simulink model "r22_05"  (Simulink 8.6)
settings: Solver=FixedStepDiscrete  StartTime=0.0  StopTime=500  FixedStep=0.1  RelTol=1e-3
undefined symbols (not defined in the file or in its folder): sldvsubsys
libraries: simulink x13, sldvlib x2
settings Model: Creator=Kerianne  LastModifiedBy=mike
settings DataIOCC: SignalLogging=off
settings OptimizationCC: DefaultParameterBehavior=Inlined
settings DebuggingCC: MultiTaskDSMMsg=warning  MultiTaskCondExecSysMsg=none  FcnCallInpInsideContextMsg=EnableAllAsError
settings GRTTargetCC: CombineOutputUpdateFcns=on  GRTInterface=off
settings ConfigComp: DVTestSuiteOptimization=CombinedObjectives (Nonlinear Extended)

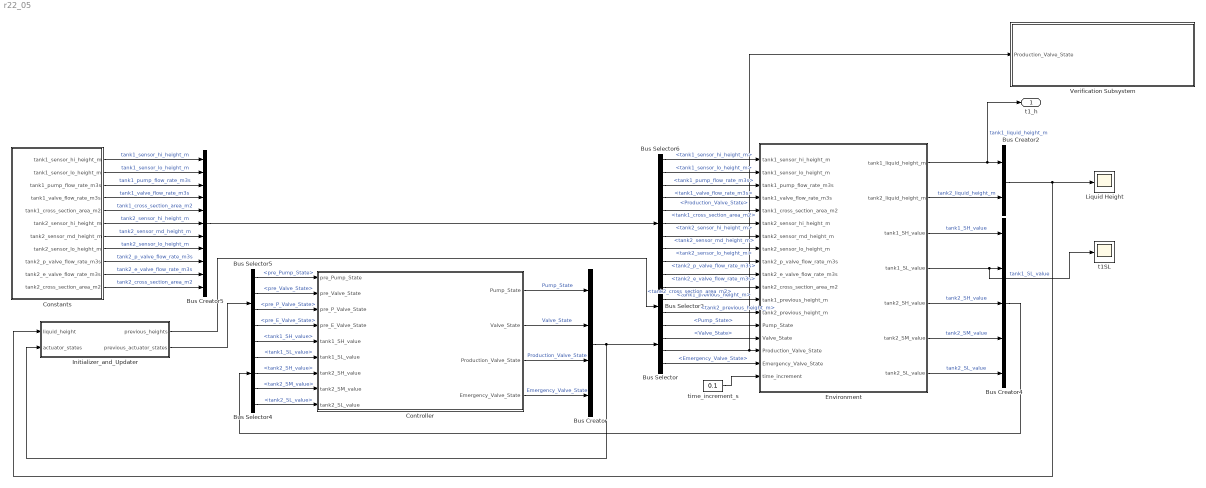
== system r22_05 ==
  Bus Creator : BusCreator  Inputs=4
  Bus Creator2 : BusCreator  Inputs='tank1_liquid_height_m','tank2_liquid_height_m'
  Bus Creator4 : BusCreator  Inputs='tank1_SH_value','tank1_SL_value','tank2_SH_value','tank2_SM_value','tank2_SL_value'
  Bus Creator5 : BusCreator  Inputs='tank1_sensor_hi_height_m','tank1_sensor_lo_height_m','tank1_pump_flow_rate_m3s','tank1_valve_flow_rate_m3s','tank1_cross_section_area_m2','tank2_sensor_hi_height_m','tank2_sensor_md_height_m','tank2_sensor_lo_height_m','tank2_p_valve_flow_rate_m3s','tank2_e_valve_flow_rate_m3s','tank2_cross_section_area_m2'
  Bus Selector : BusSelector  OutputSignals=Pump_State,Valve_State,Production_Valve_State,Emergency_Valve_State
  Bus Selector2 : BusSelector  OutputSignals=tank1_previous_height_m,tank2_previous_height_m
  Bus Selector4 : BusSelector  OutputSignals=tank1_SH_value,tank1_SL_value,tank2_SH_value,tank2_SM_value,tank2_SL_value
  Bus Selector5 : BusSelector  OutputSignals=pre_Pump_State,pre_Valve_State,pre_P_Valve_State,pre_E_Valve_State
  Bus Selector6 : BusSelector  OutputSignals=tank1_sensor_hi_height_m,tank1_sensor_lo_height_m,tank1_pump_flow_rate_m3s,tank1_valve_flow_rate_m3s,tank1_cross_section_area_m2,tank2_sensor_hi_height_m,tank2_sensor_md_height_m,tank2_sensor_lo_height_m,tank2_p_valve_flow_rate_m3s,tank2_e_valve_flow_rate_m3s,tank2_cross_section_area_m2
  Constants : Subsystem
  Controller : Subsystem
  Environment : Subsystem
  Initializer_and_Updater : Subsystem
  Liquid Height : Scope
  Verification Subsystem : Subsystem  Tag=VerificationSubsystem  DisableCoverage=on  LoadFcn=sldvsubsys('check')  TreatAsAtomicUnit=on  SimViewingDevice=on  mask(VerificationSubsystem){}
      mask init:
      | sldvsubsys('maskInit');
      settings: CopyFcn=sldvsubsys('copy');  OpenFcn=open_system(gcb,'force');
      settings: PreSaveFcn=|
      | set_param(gcb,'SimViewingDevice','on');
      | sldvsubsys('check');
      mask Help: helpview(fullfile(docroot,'toolbox','sldv','sldv.map'),'verificationsubsystem')
      mask Display: image(imread('sldvicon_versubsys.png','BackGroundColor',[1 1 1]),'center');
  t1SL : Scope
  time_increment_s : Constant  Value=0.1
  t1_h : Outport
  wires:
  Constants/1(tank1_sensor_hi_height_m) -> Bus Creator5/1  "tank1_sensor_hi_height_m"
  Constants/2(tank1_sensor_lo_height_m) -> Bus Creator5/2  "tank1_sensor_lo_height_m"
  Constants/3(tank1_pump_flow_rate_m3s) -> Bus Creator5/3  "tank1_pump_flow_rate_m3s"
  Constants/4(tank1_valve_flow_rate_m3s) -> Bus Creator5/4  "tank1_valve_flow_rate_m3s"
  Constants/5(tank1_cross_section_area_m2) -> Bus Creator5/5  "tank1_cross_section_area_m2"
  Constants/6(tank2_sensor_hi_height_m) -> Bus Creator5/6  "tank2_sensor_hi_height_m"
  Constants/7(tank2_sensor_md_height_m) -> Bus Creator5/7  "tank2_sensor_md_height_m"
  Constants/8(tank2_sensor_lo_height_m) -> Bus Creator5/8  "tank2_sensor_lo_height_m"
  Constants/9(tank2_p_valve_flow_rate_m3s) -> Bus Creator5/9  "tank2_p_valve_flow_rate_m3s"
  Constants/10(tank2_e_valve_flow_rate_m3s) -> Bus Creator5/10  "tank2_e_valve_flow_rate_m3s"
  Constants/11(tank2_cross_section_area_m2) -> Bus Creator5/11  "tank2_cross_section_area_m2"
  Controller/4(Emergency_Valve_State) -> Bus Creator/4  "Emergency_Valve_State"
  Controller/3(Production_Valve_State) -> Bus Creator/3  "Production_Valve_State"
  Controller/2(Valve_State) -> Bus Creator/2  "Valve_State"
  Controller/1(Pump_State) -> Bus Creator/1  "Pump_State"
  Bus Creator/1 -> Initializer_and_Updater/2(actuator_states), Bus Selector/1
  Bus Selector/1 -> Environment/14(Pump_State)  "<Pump_State>"
  Bus Selector/2 -> Environment/15(Valve_State)  "<Valve_State>"
  Bus Selector/3 -> Verification Subsystem/1(Production_Valve_State), Environment/16(Production_Valve_State)  "<Production_Valve_State>"
  Bus Selector/4 -> Environment/17(Emergency_Valve_State)  "<Emergency_Valve_State>"
  Environment/1(tank1_liquid_height_m) -> t1_h/1, Bus Creator2/1  "tank1_liquid_height_m"
  Environment/2(tank2_liquid_height_m) -> Bus Creator2/2  "tank2_liquid_height_m"
  Bus Selector2/1 -> Environment/12(tank1_previous_height_m)  "<tank1_previous_height_m>"
  Bus Selector2/2 -> Environment/13(tank2_previous_height_m)  "<tank2_previous_height_m>"
  Bus Creator2/1 -> Initializer_and_Updater/1(liquid_height), Liquid Height/1
  Environment/3(tank1_SH_value) -> Bus Creator4/1  "tank1_SH_value"
  Environment/4(tank1_SL_value) -> t1SL/1, Bus Creator4/2  "tank1_SL_value"
  Environment/5(tank2_SH_value) -> Bus Creator4/3  "tank2_SH_value"
  Environment/6(tank2_SM_value) -> Bus Creator4/4  "tank2_SM_value"
  Environment/7(tank2_SL_value) -> Bus Creator4/5  "tank2_SL_value"
  Bus Creator4/1 -> Bus Selector4/1
  Bus Selector5/4 -> Controller/4(pre_E_Valve_State)  "<pre_E_Valve_State>"
  Bus Selector5/1 -> Controller/1(pre_Pump_State)  "<pre_Pump_State>"
  Bus Selector5/2 -> Controller/2(pre_Valve_State)  "<pre_Valve_State>"
  Bus Selector5/3 -> Controller/3(pre_P_Valve_State)  "<pre_P_Valve_State>"
  Bus Selector4/1 -> Controller/5(tank1_SH_value)  "<tank1_SH_value>"
  Bus Selector4/2 -> Controller/6(tank1_SL_value)  "<tank1_SL_value>"
  Bus Selector4/3 -> Controller/7(tank2_SH_value)  "<tank2_SH_value>"
  Bus Selector4/4 -> Controller/8(tank2_SM_value)  "<tank2_SM_value>"
  Bus Selector4/5 -> Controller/9(tank2_SL_value)  "<tank2_SL_value>"
  Bus Creator5/1 -> Bus Selector6/1
  Bus Selector6/1 -> Environment/1(tank1_sensor_hi_height_m)  "<tank1_sensor_hi_height_m>"
  Bus Selector6/2 -> Environment/2(tank1_sensor_lo_height_m)  "<tank1_sensor_lo_height_m>"
  Bus Selector6/3 -> Environment/3(tank1_pump_flow_rate_m3s)  "<tank1_pump_flow_rate_m3s>"
  Bus Selector6/4 -> Environment/4(tank1_valve_flow_rate_m3s)  "<tank1_valve_flow_rate_m3s>"
  Bus Selector6/5 -> Environment/5(tank1_cross_section_area_m2)  "<tank1_cross_section_area_m2>"
  Bus Selector6/6 -> Environment/6(tank2_sensor_hi_height_m)  "<tank2_sensor_hi_height_m>"
  Bus Selector6/7 -> Environment/7(tank2_sensor_md_height_m)  "<tank2_sensor_md_height_m>"
  Bus Selector6/8 -> Environment/8(tank2_sensor_lo_height_m)  "<tank2_sensor_lo_height_m>"
  Bus Selector6/9 -> Environment/9(tank2_p_valve_flow_rate_m3s)  "<tank2_p_valve_flow_rate_m3s>"
  Bus Selector6/10 -> Environment/10(tank2_e_valve_flow_rate_m3s)  "<tank2_e_valve_flow_rate_m3s>"
  Bus Selector6/11 -> Environment/11(tank2_cross_section_area_m2)  "<tank2_cross_section_area_m2>"
  Initializer_and_Updater/1(previous_heights) -> Bus Selector2/1
  Initializer_and_Updater/2(previous_actuator_states) -> Bus Selector5/1
  time_increment_s/1 -> Environment/18(time_increment)

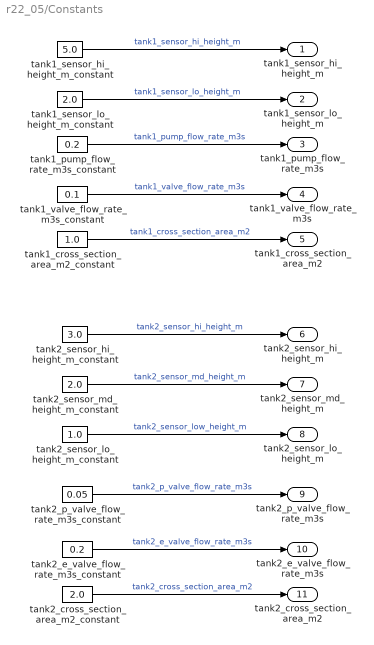
== system r22_05/Constants ==
  tank1_cross_section_area_m2_constant : Constant  Value=1.0
  tank1_pump_flow_rate_m3s_constant : Constant  Value=0.2
  tank1_sensor_hi_height_m_constant : Constant  Value=5.0
  tank1_sensor_lo_height_m_constant : Constant  Value=2.0
  tank1_valve_flow_rate_m3s_constant : Constant  Value=0.1
  tank2_cross_section_area_m2_constant : Constant  Value=2.0
  tank2_e_valve_flow_rate_m3s_constant : Constant  Value=0.2
  tank2_p_valve_flow_rate_m3s_constant : Constant  Value=0.05
  tank2_sensor_hi_height_m_constant : Constant  Value=3.0
  tank2_sensor_lo_height_m_constant : Constant  Value=1.0
  tank2_sensor_md_height_m_constant : Constant  Value=2.0
  tank1_sensor_hi_height_m : Outport
  tank1_sensor_lo_height_m : Outport  Port=2
  tank1_pump_flow_rate_m3s : Outport  Port=3
  tank1_valve_flow_rate_m3s : Outport  Port=4
  tank1_cross_section_area_m2 : Outport  Port=5
  tank2_sensor_hi_height_m : Outport  Port=6
  tank2_sensor_md_height_m : Outport  Port=7
  tank2_sensor_lo_height_m : Outport  Port=8
  tank2_p_valve_flow_rate_m3s : Outport  Port=9
  tank2_e_valve_flow_rate_m3s : Outport  Port=10
  tank2_cross_section_area_m2 : Outport  Port=11
  wires:
  tank2_sensor_hi_height_m_constant/1 -> tank2_sensor_hi_height_m/1  "tank2_sensor_hi_height_m"
  tank2_sensor_lo_height_m_constant/1 -> tank2_sensor_lo_height_m/1  "tank2_sensor_low_height_m"
  tank1_sensor_hi_height_m_constant/1 -> tank1_sensor_hi_height_m/1  "tank1_sensor_hi_height_m"
  tank1_pump_flow_rate_m3s_constant/1 -> tank1_pump_flow_rate_m3s/1  "tank1_pump_flow_rate_m3s"
  tank1_cross_section_area_m2_constant/1 -> tank1_cross_section_area_m2/1  "tank1_cross_section_area_m2"
  tank1_valve_flow_rate_m3s_constant/1 -> tank1_valve_flow_rate_m3s/1  "tank1_valve_flow_rate_m3s"
  tank1_sensor_lo_height_m_constant/1 -> tank1_sensor_lo_height_m/1  "tank1_sensor_lo_height_m"
  tank2_p_valve_flow_rate_m3s_constant/1 -> tank2_p_valve_flow_rate_m3s/1  "tank2_p_valve_flow_rate_m3s"
  tank2_cross_section_area_m2_constant/1 -> tank2_cross_section_area_m2/1  "tank2_cross_section_area_m2"
  tank2_e_valve_flow_rate_m3s_constant/1 -> tank2_e_valve_flow_rate_m3s/1  "tank2_e_valve_flow_rate_m3s"
  tank2_sensor_md_height_m_constant/1 -> tank2_sensor_md_height_m/1  "tank2_sensor_md_height_m"

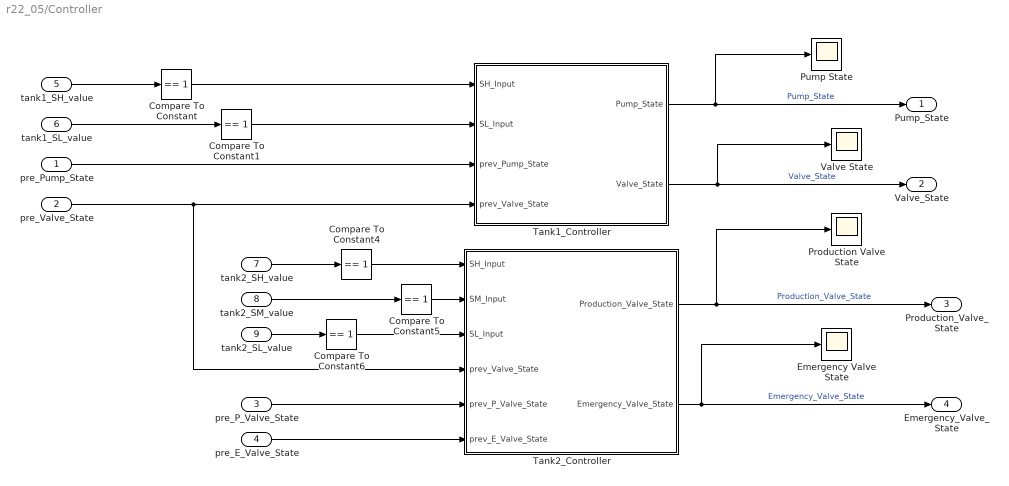
== system r22_05/Controller ==
  pre_Pump_State : Inport
  pre_Valve_State : Inport  Port=2
  pre_P_Valve_State : Inport  Port=3
  pre_E_Valve_State : Inport  Port=4
  tank1_SH_value : Inport  Port=5
  tank1_SL_value : Inport  Port=6
  tank2_SH_value : Inport  Port=7
  tank2_SM_value : Inport  Port=8
  tank2_SL_value : Inport  Port=9
  Compare To Constant{,1,4..6} (5 alike) : simulink/Logic and Bit Operations/Compare To Constant  relop===  const=1  OutDataTypeStr=boolean
  Emergency Valve State : Scope
  Production Valve State : Scope
  "Pump State " : Scope
  Tank1_Controller : Subsystem
  Tank2_Controller : Subsystem
  Valve State : Scope
  Pump_State : Outport
  Valve_State : Outport  Port=2
  Production_Valve_State : Outport  Port=3
  Emergency_Valve_State : Outport  Port=4
  wires:
  tank1_SL_value/1 -> Compare To Constant1/1
  tank2_SL_value/1 -> Compare To Constant6/1
  pre_E_Valve_State/1 -> Tank2_Controller/6(prev_E_Valve_State)
  Compare To Constant1/1 -> Tank1_Controller/2(SL_Input)
  Tank1_Controller/1(Pump_State) -> Pump_State/1, "Pump State "/1  "Pump_State"
  Tank1_Controller/2(Valve_State) -> Valve_State/1, Valve State/1  "Valve_State"
  Compare To Constant/1 -> Tank1_Controller/1(SH_Input)
  pre_Pump_State/1 -> Tank1_Controller/3(prev_Pump_State)
  tank2_SH_value/1 -> Compare To Constant4/1
  Compare To Constant6/1 -> Tank2_Controller/3(SL_Input)
  Compare To Constant4/1 -> Tank2_Controller/1(SH_Input)
  tank1_SH_value/1 -> Compare To Constant/1
  pre_Valve_State/1 -> Tank2_Controller/4(prev_Valve_State), Tank1_Controller/4(prev_Valve_State)
  Tank2_Controller/2(Emergency_Valve_State) -> Emergency_Valve_State/1, Emergency Valve State/1  "Emergency_Valve_State"
  tank2_SM_value/1 -> Compare To Constant5/1
  Compare To Constant5/1 -> Tank2_Controller/2(SM_Input)
  Tank2_Controller/1(Production_Valve_State) -> Production_Valve_State/1, Production Valve State/1  "Production_Valve_State"
  pre_P_Valve_State/1 -> Tank2_Controller/5(prev_P_Valve_State)

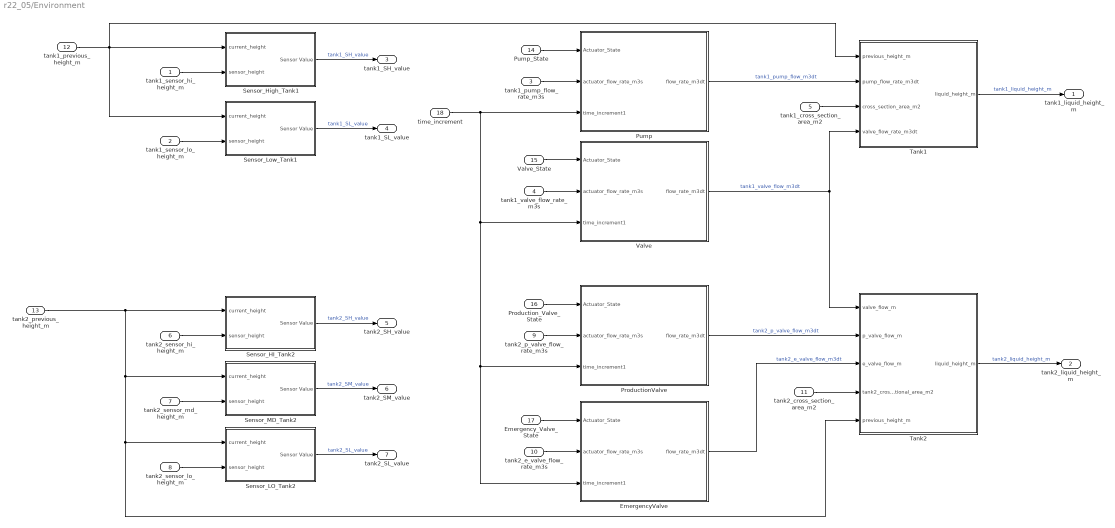
== system r22_05/Environment ==
  tank1_sensor_hi_height_m : Inport
  tank1_sensor_lo_height_m : Inport  Port=2
  tank1_pump_flow_rate_m3s : Inport  Port=3
  tank1_valve_flow_rate_m3s : Inport  Port=4
  tank1_cross_section_area_m2 : Inport  Port=5
  tank2_sensor_hi_height_m : Inport  Port=6
  tank2_sensor_md_height_m : Inport  Port=7
  tank2_sensor_lo_height_m : Inport  Port=8
  tank2_p_valve_flow_rate_m3s : Inport  Port=9
  tank2_e_valve_flow_rate_m3s : Inport  Port=10
  tank2_cross_section_area_m2 : Inport  Port=11
  tank1_previous_height_m : Inport  Port=12
  tank2_previous_height_m : Inport  Port=13
  Pump_State : Inport  Port=14
  Valve_State : Inport  Port=15
  Production_Valve_State : Inport  Port=16
  Emergency_Valve_State : Inport  Port=17
  time_increment : Inport  Port=18
  EmergencyValve : Subsystem
  ProductionValve : Subsystem
  Pump : Subsystem
  Sensor_HI_Tank2 : Subsystem
  Sensor_High_Tank1 : Subsystem
  Sensor_LO_Tank2 : Subsystem
  Sensor_Low_Tank1 : Subsystem
  Sensor_MD_Tank2 : Subsystem
  Tank1 : Subsystem
  Tank2 : Subsystem
  Valve : Subsystem
  tank1_liquid_height_m : Outport
  tank2_liquid_height_m : Outport  Port=2
  tank1_SH_value : Outport  Port=3
  tank1_SL_value : Outport  Port=4
  tank2_SH_value : Outport  Port=5
  tank2_SM_value : Outport  Port=6
  tank2_SL_value : Outport  Port=7
  wires:
  Tank1/1(liquid_height_m) -> tank1_liquid_height_m/1  "tank1_liquid_height_m"
  time_increment/1 -> Pump/3(time_increment1), Valve/3(time_increment1), EmergencyValve/3(time_increment1), ProductionValve/3(time_increment1)
  tank2_sensor_hi_height_m/1 -> Sensor_HI_Tank2/2(sensor_height)
  tank2_sensor_md_height_m/1 -> Sensor_MD_Tank2/2(sensor_height)
  Sensor_Low_Tank1/1(Sensor Value) -> tank1_SL_value/1  "tank1_SL_value"
  Sensor_HI_Tank2/1(Sensor Value) -> tank2_SH_value/1  "tank2_SH_value"
  Sensor_High_Tank1/1(Sensor Value) -> tank1_SH_value/1  "tank1_SH_value"
  tank1_pump_flow_rate_m3s/1 -> Pump/2(actuator_flow_rate_m3s)
  Sensor_LO_Tank2/1(Sensor Value) -> tank2_SL_value/1  "tank2_SL_value"
  tank2_sensor_lo_height_m/1 -> Sensor_LO_Tank2/2(sensor_height)
  tank1_valve_flow_rate_m3s/1 -> Valve/2(actuator_flow_rate_m3s)
  Sensor_MD_Tank2/1(Sensor Value) -> tank2_SM_value/1  "tank2_SM_value"
  tank2_p_valve_flow_rate_m3s/1 -> ProductionValve/2(actuator_flow_rate_m3s)
  tank2_previous_height_m/1 -> Sensor_HI_Tank2/1(current_height), Sensor_MD_Tank2/1(current_height), Tank2/5(previous_height_m), Sensor_LO_Tank2/1(current_height)
  EmergencyValve/1(flow_rate_m3dt) -> Tank2/3(e_valve_flow_m)  "tank2_e_valve_flow_m3dt"
  Pump/1(flow_rate_m3dt) -> Tank1/2(pump_flow_rate_m3dt)  "tank1_pump_flow_m3dt"
  Valve/1(flow_rate_m3dt) -> Tank2/1(valve_flow_m), Tank1/4(valve_flow_rate_m3dt)  "tank1_valve_flow_m3dt"
  ProductionValve/1(flow_rate_m3dt) -> Tank2/2(p_valve_flow_m)  "tank2_p_valve_flow_m3dt"
  tank2_e_valve_flow_rate_m3s/1 -> EmergencyValve/2(actuator_flow_rate_m3s)
  Valve_State/1 -> Valve/1(Actuator_State)
  Emergency_Valve_State/1 -> EmergencyValve/1(Actuator_State)
  Pump_State/1 -> Pump/1(Actuator_State)
  tank1_sensor_lo_height_m/1 -> Sensor_Low_Tank1/2(sensor_height)
  tank1_sensor_hi_height_m/1 -> Sensor_High_Tank1/2(sensor_height)
  Production_Valve_State/1 -> ProductionValve/1(Actuator_State)
  tank1_previous_height_m/1 -> Tank1/1(previous_height_m), Sensor_Low_Tank1/1(current_height), Sensor_High_Tank1/1(current_height)
  Tank2/1(liquid_height_m) -> tank2_liquid_height_m/1  "tank2_liquid_height_m"
  tank1_cross_section_area_m2/1 -> Tank1/3(cross_section_area_m2)
  tank2_cross_section_area_m2/1 -> Tank2/4(tank2_cross_sectional_area_m2)

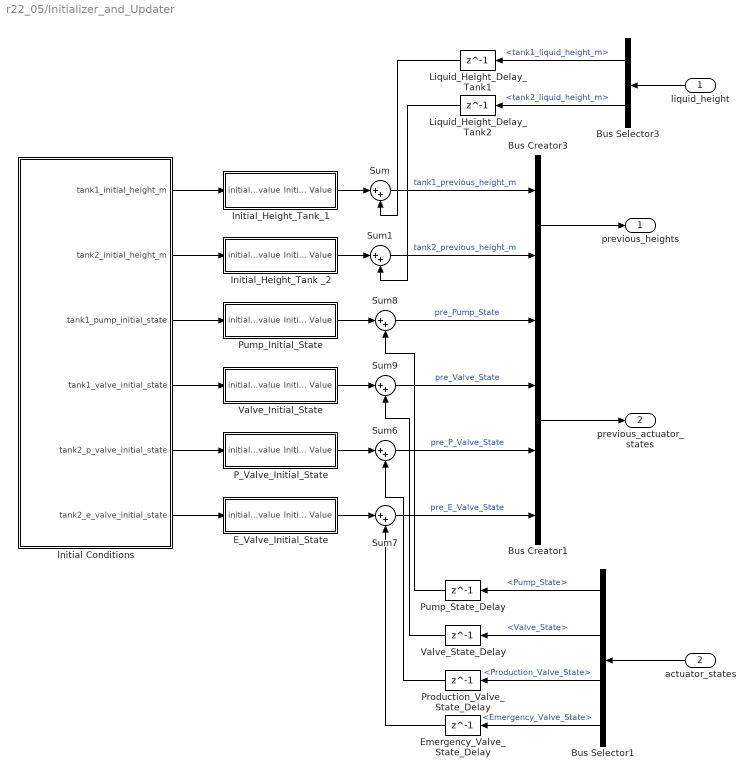
== system r22_05/Initializer_and_Updater ==
  liquid_height : Inport
  actuator_states : Inport  Port=2
  Bus Creator1 : BusCreator  Inputs='pre_Pump_State','pre_Valve_State','pre_P_Valve_State','pre_E_Valve_State'
  Bus Creator3 : BusCreator  Inputs='tank1_previous_height_m','tank2_previous_height_m'
  Bus Selector1 : BusSelector  OutputSignals=Pump_State,Valve_State,Production_Valve_State,Emergency_Valve_State
  Bus Selector3 : BusSelector  OutputSignals=tank1_liquid_height_m,tank2_liquid_height_m
  E_Valve_Initial_State : Subsystem
  Emergency_Valve_State_Delay : Delay  DelayLength=1  InitialCondition=0
  Initial Conditions : Subsystem
  Initial_Height_Tank _2 : Subsystem
  Initial_Height_Tank_1 : Subsystem
  Liquid_Height_Delay_Tank1 : Delay  DelayLength=1  InitialCondition=0
  Liquid_Height_Delay_Tank2 : Delay  DelayLength=1  InitialCondition=0
  P_Valve_Initial_State : Subsystem
  Production_Valve_State_Delay : Delay  DelayLength=1  InitialCondition=0
  Pump_Initial_State : Subsystem
  Pump_State_Delay : Delay  DelayLength=1  InitialCondition=0
  Sum{,1,6..9} (6 alike) : Sum  Inputs=|++
  Valve_Initial_State : Subsystem
  Valve_State_Delay : Delay  DelayLength=1  InitialCondition=0
  previous_heights : Outport
  previous_actuator_states : Outport  Port=2
  wires:
  Production_Valve_State_Delay/1 -> Sum6/2
  Liquid_Height_Delay_Tank1/1 -> Sum/2
  Pump_Initial_State/1(Initial Value) -> Sum8/1
  Liquid_Height_Delay_Tank2/1 -> Sum1/2
  Valve_Initial_State/1(Initial Value) -> Sum9/1
  E_Valve_Initial_State/1(Initial Value) -> Sum7/1
  Emergency_Valve_State_Delay/1 -> Sum7/2
  Bus Selector1/3 -> Production_Valve_State_Delay/1  "<Production_Valve_State>"
  Bus Selector1/1 -> Pump_State_Delay/1  "<Pump_State>"
  Bus Selector1/2 -> Valve_State_Delay/1  "<Valve_State>"
  Bus Selector1/4 -> Emergency_Valve_State_Delay/1  "<Emergency_Valve_State>"
  Initial_Height_Tank _2/1(Initial Value) -> Sum1/1
  Initial_Height_Tank_1/1(Initial Value) -> Sum/1
  Initial Conditions/3(tank1_pump_initial_state) -> Pump_Initial_State/1(initial_value)
  Initial Conditions/4(tank1_valve_initial_state) -> Valve_Initial_State/1(initial_value)
  Initial Conditions/1(tank1_initial_height_m) -> Initial_Height_Tank_1/1(initial_value)
  Initial Conditions/2(tank2_initial_height_m) -> Initial_Height_Tank _2/1(initial_value)
  Initial Conditions/5(tank2_p_valve_initial_state) -> P_Valve_Initial_State/1(initial_value)
  Initial Conditions/6(tank2_e_valve_initial_state) -> E_Valve_Initial_State/1(initial_value)
  P_Valve_Initial_State/1(Initial Value) -> Sum6/1
  Sum7/1 -> Bus Creator1/4  "pre_E_Valve_State"
  Bus Selector3/2 -> Liquid_Height_Delay_Tank2/1  "<tank2_liquid_height_m>"
  Bus Selector3/1 -> Liquid_Height_Delay_Tank1/1  "<tank1_liquid_height_m>"
  Bus Creator3/1 -> previous_heights/1
  Sum6/1 -> Bus Creator1/3  "pre_P_Valve_State"
  Sum/1 -> Bus Creator3/1  "tank1_previous_height_m"
  Sum9/1 -> Bus Creator1/2  "pre_Valve_State"
  Sum8/1 -> Bus Creator1/1  "pre_Pump_State"
  Sum1/1 -> Bus Creator3/2  "tank2_previous_height_m"
  Valve_State_Delay/1 -> Sum9/2
  Pump_State_Delay/1 -> Sum8/2
  Bus Creator1/1 -> previous_actuator_states/1
  liquid_height/1 -> Bus Selector3/1
  actuator_states/1 -> Bus Selector1/1

== system r22_05/Verification Subsystem ==
  note: Production_Valve_State{0} == 0.0;
  note: # R05 When the system is initially started the tank 2 production valve
      | # shall be CLOSED.
      | #
      | # NOTE: sensor values *should* be Boolean, BUT they are enetered as floats in the model.
  Production_Valve_State : Inport
  Compare To Constant : simulink/Logic and Bit Operations/Compare To Constant  relop===  const=0  OutDataTypeStr=boolean
  Extender : sldvlib/Temporal Operators/Extender  reset=off  ext_type=Infinite  out_hold=3
  Proof Objective1 : sldvlib/Objectives and Constraints/Proof Objective  enabled=on  customAVTBlockType=Proof Objective  intervals=true  dispValues=on  outEnabled=off  enableStopSim=off
      settings: AttributesFormatString=%<intervals>
  wires:
  Extender/1 -> Proof Objective1/1
  Production_Valve_State/1 -> Compare To Constant/1
  Compare To Constant/1 -> Extender/1

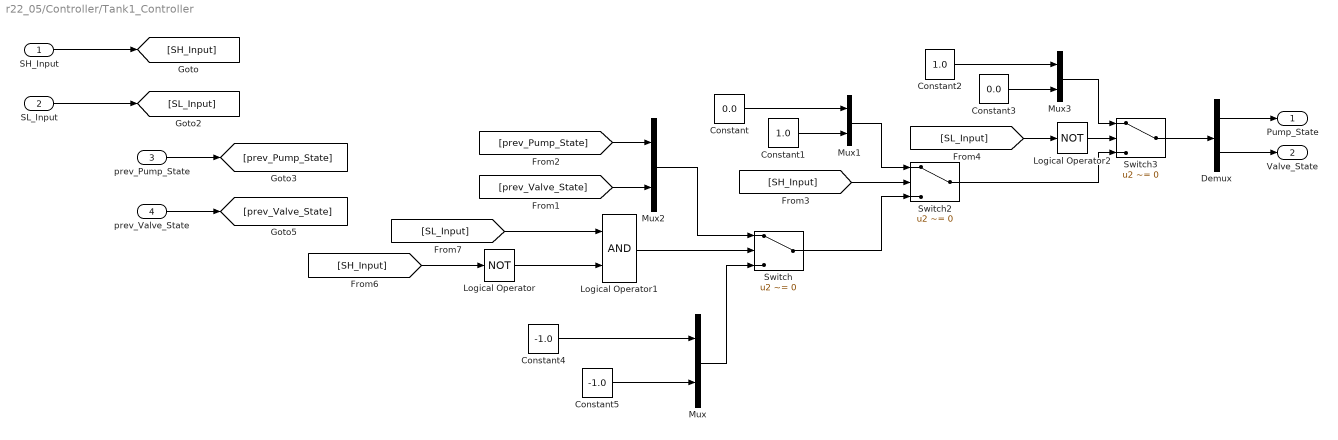
== system r22_05/Controller/Tank1_Controller ==
  SH_Input : Inport
  SL_Input : Inport  Port=2
  prev_Pump_State : Inport  Port=3
  prev_Valve_State : Inport  Port=4
  Constant : Constant  Value=0.0
  Constant1 : Constant  Value=1.0
  Constant2 : Constant  Value=1.0
  Constant3 : Constant  Value=0.0
  Constant4 : Constant  Value=-1.0
  Constant5 : Constant  Value=-1.0
  Demux : Demux  Outputs=2
  Logical Operator : Logic  Operator=NOT  AllPortsSameDT=off  OutDataTypeStr=boolean
  Logical Operator1 : Logic  AllPortsSameDT=off  OutDataTypeStr=boolean
  Logical Operator2 : Logic  Operator=NOT  AllPortsSameDT=off  OutDataTypeStr=boolean
  Mux{,1..3} (4 alike) : Mux  Inputs=2
  Switch : Switch  Criteria=u2 ~= 0
  Switch2 : Switch  Criteria=u2 ~= 0
  Switch3 : Switch  Criteria=u2 ~= 0
  Pump_State : Outport
  Valve_State : Outport  Port=2
  wires:
  prev_Pump_State/1 -> [prev_Pump_State]
  prev_Valve_State/1 -> [prev_Valve_State]
  Mux/1 -> Switch/3
  Constant/1 -> Mux1/1
  Constant1/1 -> Mux1/2
  [prev_Pump_State] -> Mux2/1
  [prev_Valve_State] -> Mux2/2
  Mux2/1 -> Switch/1
  Logical Operator1/1 -> Switch/2
  [SL_Input] -> Logical Operator1/1
  Logical Operator/1 -> Logical Operator1/2
  [SH_Input] -> Logical Operator/1
  Switch/1 -> Switch2/3
  [SH_Input] -> Switch2/2
  Mux1/1 -> Switch2/1
  [SL_Input] -> Logical Operator2/1
  Constant2/1 -> Mux3/1
  Constant3/1 -> Mux3/2
  Mux3/1 -> Switch3/1
  Switch3/1 -> Demux/1
  Demux/2 -> Valve_State/1
  SH_Input/1 -> [SH_Input]
  SL_Input/1 -> [SL_Input]
  Logical Operator2/1 -> Switch3/2
  Constant4/1 -> Mux/1
  Constant5/1 -> Mux/2
  Demux/1 -> Pump_State/1
  Switch2/1 -> Switch3/3

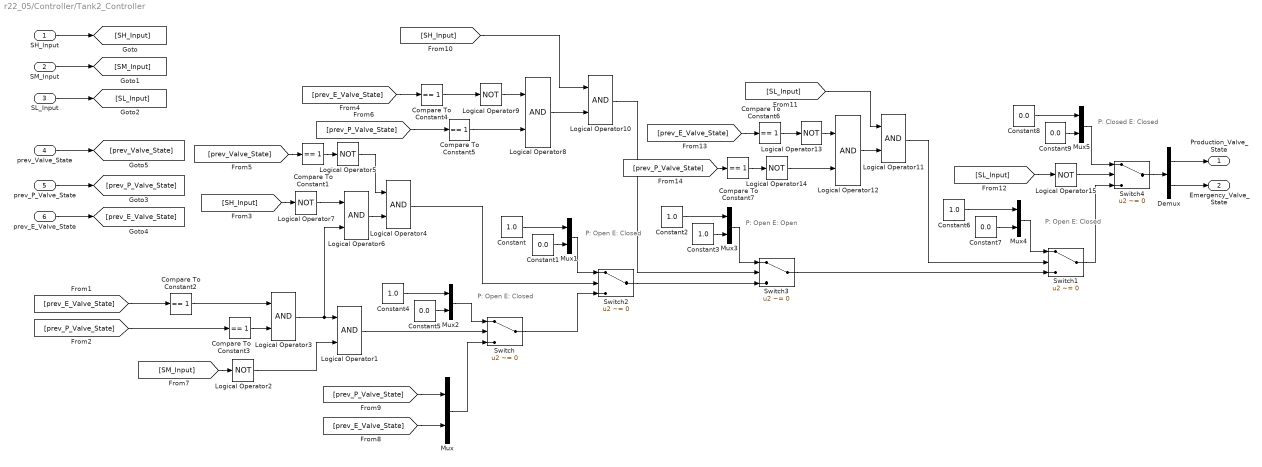
== system r22_05/Controller/Tank2_Controller ==
  note: P: Open
      | E: Closed
  note: P: Open
      | E: Closed
  note: P: Open
      | E: Open
  note: P: Open
      | E: Closed
  note: P: Closed
      | E: Closed
  SH_Input : Inport
  SM_Input : Inport  Port=2
  SL_Input : Inport  Port=3
  prev_Valve_State : Inport  Port=4
  prev_P_Valve_State : Inport  Port=5
  prev_E_Valve_State : Inport  Port=6
  Compare To Constant{1..7} (7 alike) : simulink/Logic and Bit Operations/Compare To Constant  relop===  const=1  OutDataTypeStr=boolean
  Constant{,2..4,6} (5 alike) : Constant  Value=1.0
  Constant{1,5,7..9} (5 alike) : Constant  Value=0.0
  Demux : Demux  Outputs=2
  Logical Operator{1,3..4,6,8,10..12} (8 alike) : Logic  AllPortsSameDT=off  OutDataTypeStr=boolean
  Logical Operator{2,5,7,9,13..15} (7 alike) : Logic  Operator=NOT  AllPortsSameDT=off  OutDataTypeStr=boolean
  Mux{,1..5} (6 alike) : Mux  Inputs=2
  Switch{,1..4} (5 alike) : Switch  Criteria=u2 ~= 0
  Production_Valve_State : Outport
  Emergency_Valve_State : Outport  Port=2
  wires:
  SH_Input/1 -> [SH_Input]
  SL_Input/1 -> [SL_Input]
  SM_Input/1 -> [SM_Input]
  prev_E_Valve_State/1 -> [prev_E_Valve_State]
  prev_Valve_State/1 -> [prev_Valve_State]
  prev_P_Valve_State/1 -> [prev_P_Valve_State]
  [prev_P_Valve_State] -> Mux/1
  [prev_E_Valve_State] -> Mux/2
  Mux/1 -> Switch/3
  Constant/1 -> Mux1/1
  Constant1/1 -> Mux1/2
  Logical Operator1/1 -> Switch/2
  [SM_Input] -> Logical Operator2/1
  Switch/1 -> Switch2/3
  Logical Operator4/1 -> Switch2/2
  Mux1/1 -> Switch2/1
  Switch2/1 -> Switch3/3
  Logical Operator10/1 -> Switch3/2
  Demux/1 -> Production_Valve_State/1
  Demux/2 -> Emergency_Valve_State/1
  [prev_E_Valve_State] -> Compare To Constant2/1
  [prev_P_Valve_State] -> Compare To Constant3/1
  [prev_Valve_State] -> Compare To Constant1/1
  Logical Operator5/1 -> Logical Operator4/1
  Logical Operator6/1 -> Logical Operator4/2
  Logical Operator3/1 -> Logical Operator6/2, Logical Operator1/1
  Logical Operator2/1 -> Logical Operator1/2
  [SH_Input] -> Logical Operator7/1
  Logical Operator7/1 -> Logical Operator6/1
  Constant4/1 -> Mux2/1
  Constant5/1 -> Mux2/2
  Mux2/1 -> Switch/1
  [prev_E_Valve_State] -> Compare To Constant4/1
  [prev_P_Valve_State] -> Compare To Constant5/1
  Logical Operator9/1 -> Logical Operator8/1
  Logical Operator8/1 -> Logical Operator10/2
  Constant2/1 -> Mux3/1
  Constant3/1 -> Mux3/2
  Mux3/1 -> Switch3/1
  [prev_E_Valve_State] -> Compare To Constant6/1
  [prev_P_Valve_State] -> Compare To Constant7/1
  Logical Operator13/1 -> Logical Operator12/1
  Logical Operator12/1 -> Logical Operator11/2
  [SL_Input] -> Logical Operator11/1
  Logical Operator14/1 -> Logical Operator12/2
  Switch3/1 -> Switch1/3
  Logical Operator11/1 -> Switch1/2
  Constant6/1 -> Mux4/1
  Constant7/1 -> Mux4/2
  Mux4/1 -> Switch1/1
  Switch1/1 -> Switch4/3
  Logical Operator15/1 -> Switch4/2
  [SL_Input] -> Logical Operator15/1
  Switch4/1 -> Demux/1
  Constant8/1 -> Mux5/1
  Constant9/1 -> Mux5/2
  Mux5/1 -> Switch4/1
  [SH_Input] -> Logical Operator10/1
  Compare To Constant1/1 -> Logical Operator5/1
  Compare To Constant2/1 -> Logical Operator3/1
  Compare To Constant3/1 -> Logical Operator3/2
  Compare To Constant4/1 -> Logical Operator9/1
  Compare To Constant5/1 -> Logical Operator8/2
  Compare To Constant6/1 -> Logical Operator13/1
  Compare To Constant7/1 -> Logical Operator14/1

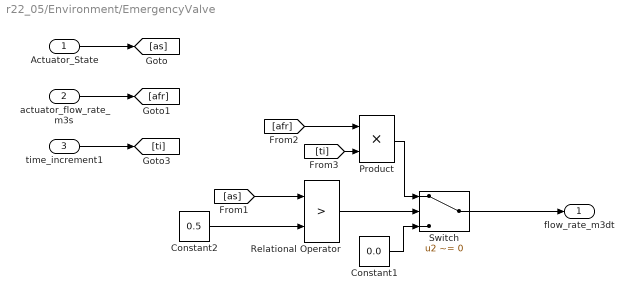
== system r22_05/Environment/EmergencyValve ==
  Actuator_State : Inport
  actuator_flow_rate_m3s : Inport  Port=2
  time_increment1 : Inport  Port=3
  Constant1 : Constant  Value=0.0
  Constant2 : Constant  Value=0.5
  Product : Product
  Relational Operator : RelationalOperator  Operator=>  OutDataTypeStr=boolean
  Switch : Switch  Criteria=u2 ~= 0
  flow_rate_m3dt : Outport
  wires:
  Relational Operator/1 -> Switch/2
  [as] -> Relational Operator/1
  [ti] -> Product/2
  Constant1/1 -> Switch/3
  Constant2/1 -> Relational Operator/2
  Actuator_State/1 -> [as]
  actuator_flow_rate_m3s/1 -> [afr]
  Switch/1 -> flow_rate_m3dt/1
  Product/1 -> Switch/1
  time_increment1/1 -> [ti]
  [afr] -> Product/1

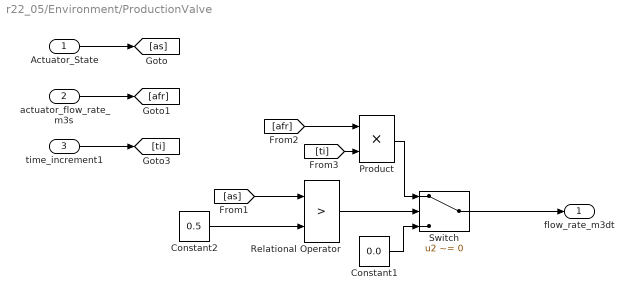
== system r22_05/Environment/ProductionValve ==
  Actuator_State : Inport
  actuator_flow_rate_m3s : Inport  Port=2
  time_increment1 : Inport  Port=3
  Constant1 : Constant  Value=0.0
  Constant2 : Constant  Value=0.5
  Product : Product
  Relational Operator : RelationalOperator  Operator=>  OutDataTypeStr=boolean
  Switch : Switch  Criteria=u2 ~= 0
  flow_rate_m3dt : Outport
  wires:
  [afr] -> Product/1
  time_increment1/1 -> [ti]
  Product/1 -> Switch/1
  Switch/1 -> flow_rate_m3dt/1
  actuator_flow_rate_m3s/1 -> [afr]
  Actuator_State/1 -> [as]
  Constant2/1 -> Relational Operator/2
  Constant1/1 -> Switch/3
  [ti] -> Product/2
  [as] -> Relational Operator/1
  Relational Operator/1 -> Switch/2

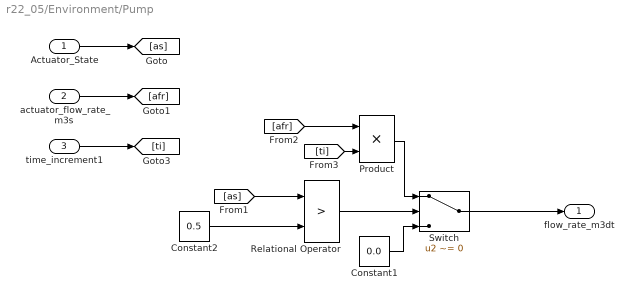
== system r22_05/Environment/Pump ==
  Actuator_State : Inport
  actuator_flow_rate_m3s : Inport  Port=2
  time_increment1 : Inport  Port=3
  Constant1 : Constant  Value=0.0
  Constant2 : Constant  Value=0.5
  Product : Product
  Relational Operator : RelationalOperator  Operator=>  OutDataTypeStr=boolean
  Switch : Switch  Criteria=u2 ~= 0
  flow_rate_m3dt : Outport
  wires:
  [afr] -> Product/1
  time_increment1/1 -> [ti]
  Product/1 -> Switch/1
  Switch/1 -> flow_rate_m3dt/1
  actuator_flow_rate_m3s/1 -> [afr]
  Actuator_State/1 -> [as]
  Constant2/1 -> Relational Operator/2
  Constant1/1 -> Switch/3
  [ti] -> Product/2
  [as] -> Relational Operator/1
  Relational Operator/1 -> Switch/2

== system r22_05/Environment/Sensor_HI_Tank2 ==
  current_height : Inport
  sensor_height : Inport  Port=2
  Constant : Constant  Value=0.0
  Constant1 : Constant  Value=1.0
  Relational Operator : RelationalOperator  Operator=>  OutDataTypeStr=boolean
  Switch : Switch  Criteria=u2 ~= 0
  Sensor Value : Outport
  wires:
  Constant/1 -> Switch/1
  sensor_height/1 -> [sh]
  [sh] -> Relational Operator/1
  Constant1/1 -> Switch/3
  Relational Operator/1 -> Switch/2
  current_height/1 -> [ch]
  [ch] -> Relational Operator/2
  Switch/1 -> Sensor Value/1

== system r22_05/Environment/Sensor_High_Tank1 ==
  current_height : Inport
  sensor_height : Inport  Port=2
  Constant : Constant  Value=0.0
  Constant1 : Constant  Value=1.0
  Relational Operator : RelationalOperator  Operator=>  OutDataTypeStr=boolean
  Switch : Switch  Criteria=u2 ~= 0
  Sensor Value : Outport
  wires:
  Constant/1 -> Switch/1
  sensor_height/1 -> [sh]
  [sh] -> Relational Operator/1
  Constant1/1 -> Switch/3
  Relational Operator/1 -> Switch/2
  current_height/1 -> [ch]
  [ch] -> Relational Operator/2
  Switch/1 -> Sensor Value/1

== system r22_05/Environment/Sensor_LO_Tank2 ==
  current_height : Inport
  sensor_height : Inport  Port=2
  Constant : Constant  Value=0.0
  Constant1 : Constant  Value=1.0
  Relational Operator : RelationalOperator  Operator=>  OutDataTypeStr=boolean
  Switch : Switch  Criteria=u2 ~= 0
  Sensor Value : Outport
  wires:
  Constant/1 -> Switch/1
  sensor_height/1 -> [sh]
  [sh] -> Relational Operator/1
  Constant1/1 -> Switch/3
  Relational Operator/1 -> Switch/2
  current_height/1 -> [ch]
  [ch] -> Relational Operator/2
  Switch/1 -> Sensor Value/1

== system r22_05/Environment/Sensor_Low_Tank1 ==
  current_height : Inport
  sensor_height : Inport  Port=2
  Constant : Constant  Value=0.0
  Constant1 : Constant  Value=1.0
  Relational Operator : RelationalOperator  Operator=>  OutDataTypeStr=boolean
  Switch : Switch  Criteria=u2 ~= 0
  Sensor Value : Outport
  wires:
  Switch/1 -> Sensor Value/1
  [ch] -> Relational Operator/2
  current_height/1 -> [ch]
  Relational Operator/1 -> Switch/2
  Constant1/1 -> Switch/3
  [sh] -> Relational Operator/1
  sensor_height/1 -> [sh]
  Constant/1 -> Switch/1

== system r22_05/Environment/Sensor_MD_Tank2 ==
  current_height : Inport
  sensor_height : Inport  Port=2
  Constant : Constant  Value=0.0
  Constant1 : Constant  Value=1.0
  Relational Operator : RelationalOperator  Operator=>  OutDataTypeStr=boolean
  Switch : Switch  Criteria=u2 ~= 0
  Sensor Value : Outport
  wires:
  Switch/1 -> Sensor Value/1
  [ch] -> Relational Operator/2
  current_height/1 -> [ch]
  Relational Operator/1 -> Switch/2
  Constant1/1 -> Switch/3
  [sh] -> Relational Operator/1
  sensor_height/1 -> [sh]
  Constant/1 -> Switch/1

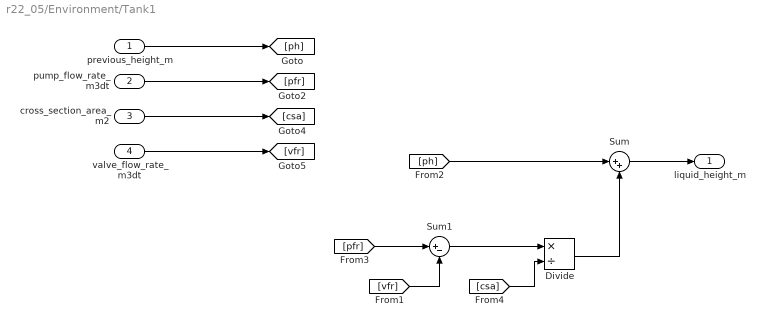
== system r22_05/Environment/Tank1 ==
  previous_height_m : Inport
  pump_flow_rate_m3dt : Inport  Port=2
  cross_section_area_m2 : Inport  Port=3
  valve_flow_rate_m3dt : Inport  Port=4
  Divide : Product  Inputs=*/
  Sum : Sum  Inputs=|++
  Sum1 : Sum  Inputs=|+-
  liquid_height_m : Outport
  wires:
  Sum/1 -> liquid_height_m/1
  cross_section_area_m2/1 -> [csa]
  [ph] -> Sum/1
  Divide/1 -> Sum/2
  valve_flow_rate_m3dt/1 -> [vfr]
  [csa] -> Divide/2
  Sum1/1 -> Divide/1
  previous_height_m/1 -> [ph]
  [vfr] -> Sum1/2
  pump_flow_rate_m3dt/1 -> [pfr]
  [pfr] -> Sum1/1

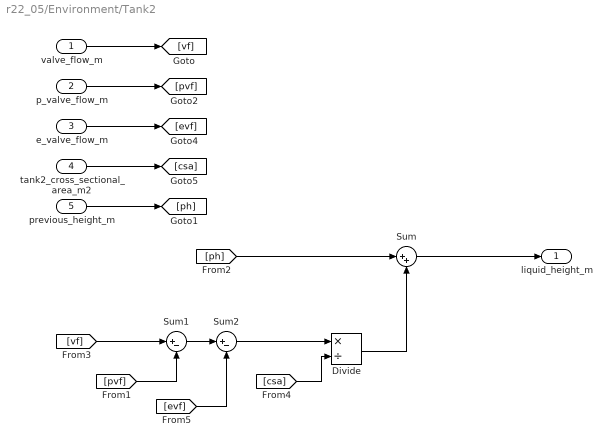
== system r22_05/Environment/Tank2 ==
  valve_flow_m : Inport
  p_valve_flow_m : Inport  Port=2
  e_valve_flow_m : Inport  Port=3
  tank2_cross_sectional_area_m2 : Inport  Port=4
  previous_height_m : Inport  Port=5
  Divide : Product  Inputs=*/
  Sum : Sum  Inputs=|++
  Sum1 : Sum  Inputs=|+-
  Sum2 : Sum  Inputs=|+-
  liquid_height_m : Outport
  wires:
  [evf] -> Sum2/2
  valve_flow_m/1 -> [vf]
  Sum/1 -> liquid_height_m/1
  p_valve_flow_m/1 -> [pvf]
  Divide/1 -> Sum/2
  [csa] -> Divide/2
  [ph] -> Sum/1
  tank2_cross_sectional_area_m2/1 -> [csa]
  previous_height_m/1 -> [ph]
  [vf] -> Sum1/1
  e_valve_flow_m/1 -> [evf]
  Sum2/1 -> Divide/1
  [pvf] -> Sum1/2
  Sum1/1 -> Sum2/1

== system r22_05/Environment/Valve ==
  Actuator_State : Inport
  actuator_flow_rate_m3s : Inport  Port=2
  time_increment1 : Inport  Port=3
  Constant1 : Constant  Value=0.0
  Constant2 : Constant  Value=0.5
  Product : Product
  Relational Operator : RelationalOperator  Operator=>  OutDataTypeStr=boolean
  Switch : Switch  Criteria=u2 ~= 0
  flow_rate_m3dt : Outport
  wires:
  Relational Operator/1 -> Switch/2
  [as] -> Relational Operator/1
  [ti] -> Product/2
  Constant1/1 -> Switch/3
  Constant2/1 -> Relational Operator/2
  Actuator_State/1 -> [as]
  actuator_flow_rate_m3s/1 -> [afr]
  Switch/1 -> flow_rate_m3dt/1
  Product/1 -> Switch/1
  time_increment1/1 -> [ti]
  [afr] -> Product/1

== system r22_05/Initializer_and_Updater/E_Valve_Initial_State ==
  initial_value : Inport
  Constant : Constant  Value=0.0
  Switch : Switch  Criteria=u2 > Threshold
  Unit Delay : UnitDelay  InitialCondition=1  SampleTime=-1
  Initial Value : Outport
  wires:
  Switch/1 -> Initial Value/1
  Constant/1 -> Switch/3, Unit Delay/1
  Unit Delay/1 -> Switch/2
  initial_value/1 -> Switch/1

== system r22_05/Initializer_and_Updater/Initial Conditions ==
  tank1_init_height_m : Constant  Value=0.0
  tank1_pump_init_state : Constant  Value=0.0
  tank1_valve_init_state : Constant  Value=0.0
  tank2_e_valve_init_state : Constant  Value=0.0
  tank2_init_height_m : Constant  Value=0.0
  tank2_p_valve_init_state : Constant  Value=0.0
  tank1_initial_height_m : Outport
  tank2_initial_height_m : Outport  Port=2
  tank1_pump_initial_state : Outport  Port=3
  tank1_valve_initial_state : Outport  Port=4
  tank2_p_valve_initial_state : Outport  Port=5
  tank2_e_valve_initial_state : Outport  Port=6
  wires:
  tank1_pump_init_state/1 -> tank1_pump_initial_state/1  "tank1_pump_initial_state"
  tank2_e_valve_init_state/1 -> tank2_e_valve_initial_state/1  "tank2_e_valve_initial_state"
  tank2_p_valve_init_state/1 -> tank2_p_valve_initial_state/1  "tank2_p_valve_initial_state"
  tank1_init_height_m/1 -> tank1_initial_height_m/1  "tank1_initial_height_m"
  tank2_init_height_m/1 -> tank2_initial_height_m/1  "tank2_initial_height_m"
  tank1_valve_init_state/1 -> tank1_valve_initial_state/1  "tank1_valve_initial_state"

== system r22_05/Initializer_and_Updater/Initial_Height_Tank _2 ==
  initial_value : Inport
  Constant : Constant  Value=0.0
  Switch : Switch  Criteria=u2 > Threshold
  Unit Delay : UnitDelay  InitialCondition=1  SampleTime=-1
  Initial Value : Outport
  wires:
  Switch/1 -> Initial Value/1
  Constant/1 -> Switch/3, Unit Delay/1
  Unit Delay/1 -> Switch/2
  initial_value/1 -> Switch/1

== system r22_05/Initializer_and_Updater/Initial_Height_Tank_1 ==
  initial_value : Inport
  Constant : Constant  Value=0.0
  Switch : Switch  Criteria=u2 > Threshold
  Unit Delay : UnitDelay  InitialCondition=1  SampleTime=-1
  Initial Value : Outport
  wires:
  Switch/1 -> Initial Value/1
  Constant/1 -> Switch/3, Unit Delay/1
  Unit Delay/1 -> Switch/2
  initial_value/1 -> Switch/1

== system r22_05/Initializer_and_Updater/P_Valve_Initial_State ==
  initial_value : Inport
  Constant : Constant  Value=0.0
  Switch : Switch  Criteria=u2 > Threshold
  Unit Delay : UnitDelay  InitialCondition=1  SampleTime=-1
  Initial Value : Outport
  wires:
  Switch/1 -> Initial Value/1
  Constant/1 -> Switch/3, Unit Delay/1
  Unit Delay/1 -> Switch/2
  initial_value/1 -> Switch/1

== system r22_05/Initializer_and_Updater/Pump_Initial_State ==
  initial_value : Inport
  Constant : Constant  Value=0.0
  Switch : Switch  Criteria=u2 > Threshold
  Unit Delay : UnitDelay  InitialCondition=1  SampleTime=-1
  Initial Value : Outport
  wires:
  Switch/1 -> Initial Value/1
  Constant/1 -> Switch/3, Unit Delay/1
  Unit Delay/1 -> Switch/2
  initial_value/1 -> Switch/1

== system r22_05/Initializer_and_Updater/Valve_Initial_State ==
  initial_value : Inport
  Constant : Constant  Value=0.0
  Switch : Switch  Criteria=u2 > Threshold
  Unit Delay : UnitDelay  InitialCondition=1  SampleTime=-1
  Initial Value : Outport
  wires:
  Switch/1 -> Initial Value/1
  Constant/1 -> Switch/3, Unit Delay/1
  Unit Delay/1 -> Switch/2
  initial_value/1 -> Switch/1
